simulink model "ex00_model"  (R2023a)
settings: Solver=FixedStepDiscrete  StartTime=0.0  StopTime=10000*Ts  RelTol=1e-3
undefined symbols (not defined in the file): Fc, h, h_matrix, L, Ts
libraries: dspsigops x3, dspsrcs4 x2
settings Model: Creator=daniele  LastModifiedBy=mluser
settings SolverCC: AlgebraicLoopSolver=TrustRegion
settings DataIOCC: ReturnWorkspaceOutputs=off
settings DebuggingCC: UnconnectedInputMsg=warning  UnconnectedOutputMsg=warning  UnconnectedLineMsg=warning  ArithmeticOperatorsInVariantConditions=warning
settings ModelReferenceCC: EnableRefExpFcnMdlSchedulingChecks=on
settings SFSimCC: CustomCodeUndefinedFunction=UseInterfaceOnly

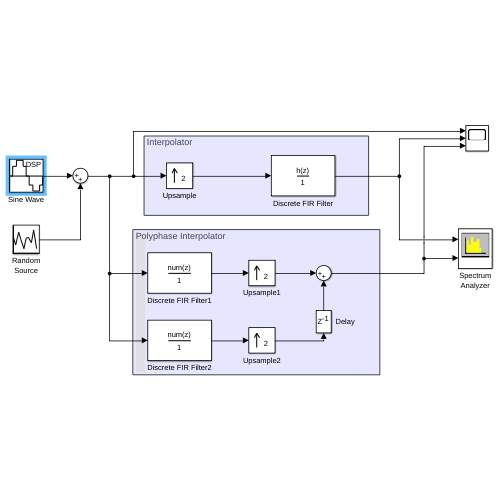
[thumbnail: Simulink's stored preview of the top-level diagram]
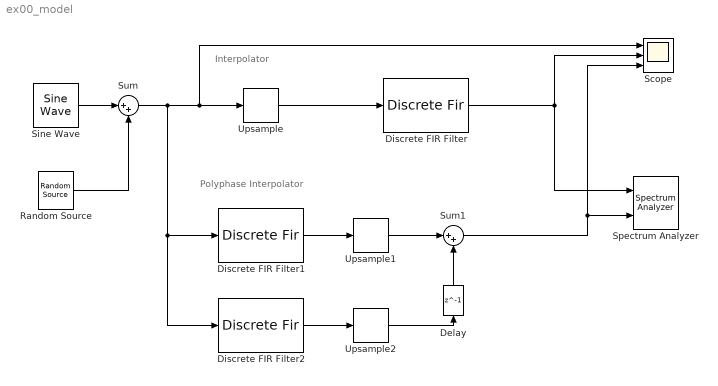
== system ex00_model ==
  note: Polyphase Interpolator
  note: Interpolator
  Delay : Delay  DelayLength=1  InitialCondition=0  UseCircularBuffer=on
  Discrete FIR Filter : DiscreteFir  Coefficients=h
  Discrete FIR Filter1 : DiscreteFir  Coefficients=h_matrix(1,:)
  Discrete FIR Filter2 : DiscreteFir  Coefficients=h_matrix(2,:)
  Random Source : dspsrcs4/Random Source  SrcType=Gaussian  NormMethod=Ziggurat  CltLength=12  MinVal=0  MaxVal=1  MeanVal=0  VarVal=0.5  RepMode=Not repeatable  rawSeed=1  IsInherit=off  SampMode=Discrete  SampTime=Ts  SampFrame=1  DataType=Double  OutComplex=Real  OutputFrames=off
  Scope : Scope  NumInputPorts=3
  Sine Wave : dspsrcs4/Sine Wave  Amplitude=1  Frequency=Fc  Phase=0  SampleMode=Discrete  OutComplex=Real  CompMethod=Trigonometric fcn  TableSize=Speed  SampleTime=Ts  SamplesPerFrame=1  ResetState=Restart at time zero  OutputFrames=off  dataType=double  wordLen=16  udDataType=sfix(16)  fracBitsMode=Best precision  numFracBits=15  OutDataTypeStr=double  LastOutDataTypeStr=double
  Spectrum Analyzer : SpectrumAnalyzer  NumInputPorts=2  WindowPosition=[199.000000,88.000000,800.000000,500.000000,]  ScopeFrameLocation=window  YLimits=[-113.33275089,31.5987389]  ColorLimits=[-20 80]  ShowLegend=on  SelectedToolstripTab=spectrumAnalyzerToolstrip.measurementsTab  DefaultConfigurationName=spbscopes.SpectrumAnalyzerBlockCfg  IsFrequencyInputMode=0  FrequencyVectorPort=0  FrequencyVectorFromPort=0  FrequencyInputRBWPort=0  FrequencyInputRBWFromPort=0
  Sum : Sum  Inputs=|++
  Sum1 : Sum  Inputs=|++
  Upsample : dspsigops/Upsample  FactorSource=Dialog parameter  N=L  Nmax=16  phase=0  RateOptions=Allow multirate processing  ic=0  mode=Unused parameter value
      settings: LibrarySourceBlock=dsphdlsupportsigops/Upsample
  Upsample1 : dspsigops/Upsample  FactorSource=Dialog parameter  N=L  Nmax=16  phase=0  RateOptions=Allow multirate processing  ic=0  mode=Unused parameter value
      settings: LibrarySourceBlock=dsphdlsupportsigops/Upsample
  Upsample2 : dspsigops/Upsample  FactorSource=Dialog parameter  N=L  Nmax=16  phase=0  RateOptions=Allow multirate processing  ic=0  mode=Unused parameter value
      settings: LibrarySourceBlock=dsphdlsupportsigops/Upsample
  wires:
  Sine Wave/1 -> Sum/1
  Random Source/1 -> Sum/2
  Sum/1 -> Discrete FIR Filter2/1, Discrete FIR Filter1/1, Scope/1, Upsample/1
  Upsample/1 -> Discrete FIR Filter/1
  Discrete FIR Filter1/1 -> Upsample1/1
  Discrete FIR Filter2/1 -> Upsample2/1
  Upsample1/1 -> Sum1/1
  Upsample2/1 -> Delay/1
  Delay/1 -> Sum1/2
  Sum1/1 -> Scope/3, Spectrum Analyzer/2
  Discrete FIR Filter/1 -> Spectrum Analyzer/1, Scope/2
